simulink model "SolarTrackerHardwareModel"  (R2020a)
settings: Solver=FixedStepAuto  StartTime=0.0  StopTime=10.0  RelTol=1e-3
undefined symbols (not defined in the file): Fi, Wi
libraries: arduinowifilib x5, arduinolib x2, simulink x2
settings Model: SILPILModeSetting=veronly  ExtModeTrigDuration=2  Creator=cstap  LastModifiedBy=cstapels
settings OptimizationCC: EnhancedBackFolding=on  PassReuseOutputArgsAs=Individual arguments  ZeroExternalMemoryAtStartup=off  ZeroInternalMemoryAtStartup=off  MaxStackSize=64  OptimizeBlockOrder=speed  DifferentSizesBufferReuse=on  OptimizationCustomize=off  EfficientTunableParamExpr=on
settings DebuggingCC: ParameterTunabilityLossMsg=error
settings HardwareCC: ProdBitPerPointer=32  ProdBitPerSizeT=32  ProdBitPerPtrDiffT=32  ProdLargestAtomicInteger=Long  ProdLargestAtomicFloat=Double  ProdWordSize=32  ProdHWDeviceType=ARM Compatible->ARM Cortex
settings SFSimCC: MATLABDynamicMemAlloc=off
settings RTWCC: SystemTargetFile=ert.tlc  HardwareBoard=Arduino MKR1000  TLCOptions=-aInlineSetEventsForThisBaseRateFcn=TLC_FALSE -aSuppressMultiTaskScheduler=TLC_FALSE -aRateBasedStepFcn=1  TemplateMakefile=ert_default_tmf  Toolchain=Arduino ARM  BuildConfiguration=Faster Runs
settings CodeAppCC: ForceParamTrailComments=on  IgnoreCustomStorageClasses=off  OperatorAnnotations=on  SimulinkDataObjDesc=on  SFDataObjDesc=on  InsertBlockDesc=on
settings ERTTargetCC: SupportContinuousTime=on  SupportVariableSizeSignals=on  ExtModeStaticAllocSize=8192

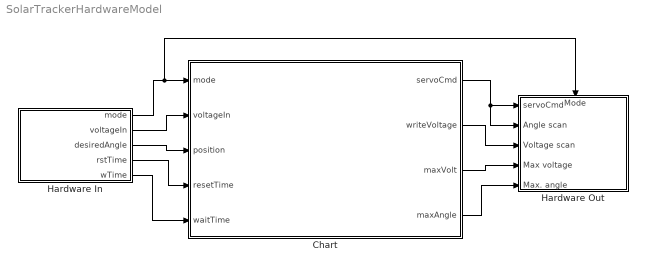
== system SolarTrackerHardwareModel ==
  Chart : Stateflow chart  TreatAsAtomicUnit=on
      settings: PortSchema="{\"entries\":[{\"content\":{\"sides\":[{\"content\":{\"connectorIds\":[\"In5\",\"In1\",\"In2\",\"In3\",\"In4\"]},\"type\":\"ConnectorPlacement.EquallySpacedRectSide\",\"uuid\":\"7460febf-f6e8-4dab-9ef6-8acf957c7b17\"},{\"content\":{\"connectorIds\":[\"Out1\",\"Out2\",\"Out3\",\"Out4\"],\"side\":\"RIGHT\"},\"type\":\"ConnectorPlacement.EquallySpacedRectSide\",\"uuid\":\"34f4fde0-3abd-4f83-b5ac-d115b7860e10\"},{\"content\":{\"connectorIds\":[],\"side\":\"TOP\"},\"type\":\"ConnectorPlacement.EquallySpacedRectSide\",\"uuid\":\"03c52414-b361-422d-a974-9760757eaedc\"}]},\"type\":\"ConnectorPlacement.EquallySpacedConnector\",\"uuid\":\"cf5b2fd0-3883-4494-a5b1-8c312db57bd7\"}],\"packageUris\":[\"http://schema.mathworks.com/mf0/Connector/19700101\"],\"version\":\"1.0\"}"
  Hardware In : Subsystem  VariantControl=simulationMode == 0
  Hardware Out : Subsystem  VariantControl=simulationMode == 0
      settings: PortSchema="{\"entries\":[{\"content\":{\"sides\":[{\"content\":{\"connectorIds\":[\"In1\",\"In2\",\"In3\",\"In4\",\"In5\"]},\"type\":\"ConnectorPlacement.EquallySpacedRectSide\",\"uuid\":\"deada059-bee1-4c5a-83e8-1a3ffab69375\"},{\"content\":{\"connectorIds\":[],\"side\":\"RIGHT\"},\"type\":\"ConnectorPlacement.EquallySpacedRectSide\",\"uuid\":\"cbd49981-471a-4624-8e3d-3b37af600932\"},{\"content\":{\"connectorIds\":[\"In6\"],\"side\":\"TOP\"},\"type\":\"ConnectorPlacement.EquallySpacedRectSide\",\"uuid\":\"9a45ed85-a60b-4cc5-836b-a1fc991137ba\"}]},\"type\":\"ConnectorPlacement.EquallySpacedConnector\",\"uuid\":\"2ce86ef1-c832-4a6c-ba54-7fb04718268c\"}],\"packageUris\":[\"http://schema.mathworks.com/mf0/Connector/19700101\"],\"version\":\"1.0\"}"
  wires:
  Hardware In/1(mode) -> Hardware Out/6(Mode), Chart/5(mode)
  Hardware In/2(voltageIn) -> Chart/1(voltageIn)
  Hardware In/3(desiredAngle) -> Chart/2(position)
  Hardware In/4(rstTime) -> Chart/3(resetTime)
  Hardware In/5(wTime) -> Chart/4(waitTime)
  Chart/1(servoCmd) -> Hardware Out/2(Angle scan), Hardware Out/1(servoCmd)
  Chart/2(writeVoltage) -> Hardware Out/3(Voltage scan)
  Chart/3(maxVolt) -> Hardware Out/4(Max voltage)
  Chart/4(maxAngle) -> Hardware Out/5(Max. angle)

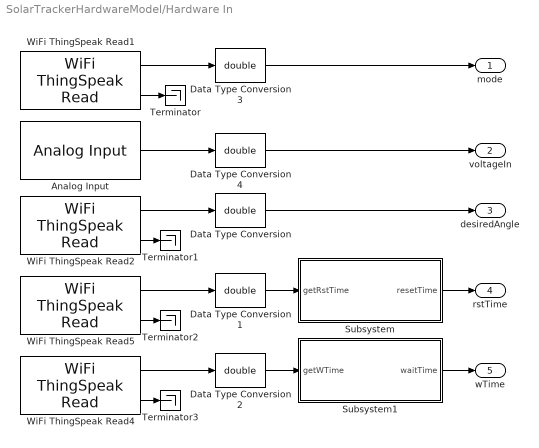
== system SolarTrackerHardwareModel/Hardware In ==
  Analog Input : arduinolib/Analog Input  pinNumber=1  ReadResultsOnly=off  ConversionTriggerSource=Software  ExternalTriggerType=uint32( 0 )  OutputDataType=uint16  EnableConversionCompleteNotify=off  EnableOuputStatus=off  SampleTime=-1  blockPlatform=arduino
  Data Type Conversion{,1..4} (5 alike) : DataTypeConversion  OutDataTypeStr=double
  Subsystem : Subsystem
  Subsystem1 : Subsystem
  Terminator{,1..3} (4 alike) : Terminator
  WiFi ThingSpeak Read1 : arduinowifilib/WiFi ThingSpeak Read  ChannelID_=1005403  ChannelAccess_=Private  ReadAPIKey_=RTAKGVYMGG3OII72  FieldNumber_=1  PrintDiagnosticMessages_=off  blockPlatform=Arduino  Interfacetype_=Wi-Fi  SampleTime_=30
      settings: SourceProductBaseCode=ARDUINO
  WiFi ThingSpeak Read2 : arduinowifilib/WiFi ThingSpeak Read  ChannelID_=1005403  ChannelAccess_=Private  ReadAPIKey_=RTAKGVYMGG3OII72  FieldNumber_=2  PrintDiagnosticMessages_=off  blockPlatform=Arduino  Interfacetype_=Wi-Fi  SampleTime_=30
      settings: SourceProductBaseCode=ARDUINO
  WiFi ThingSpeak Read4 : arduinowifilib/WiFi ThingSpeak Read  ChannelID_=1005403  ChannelAccess_=Private  ReadAPIKey_=RTAKGVYMGG3OII72  FieldNumber_=4  PrintDiagnosticMessages_=off  blockPlatform=Arduino  Interfacetype_=Wi-Fi  SampleTime_=30
      settings: SourceProductBaseCode=ARDUINO
  WiFi ThingSpeak Read5 : arduinowifilib/WiFi ThingSpeak Read  ChannelID_=1005403  ChannelAccess_=Private  ReadAPIKey_=RTAKGVYMGG3OII72  FieldNumber_=3  PrintDiagnosticMessages_=off  blockPlatform=Arduino  Interfacetype_=Wi-Fi  SampleTime_=30
      settings: SourceProductBaseCode=ARDUINO
  mode : Outport
  voltageIn : Outport  Port=2
  desiredAngle : Outport  Port=3
  rstTime : Outport  Port=4
  wTime : Outport  Port=5
  wires:
  WiFi ThingSpeak Read1/2 -> Terminator/1
  Subsystem/1(resetTime) -> rstTime/1
  Subsystem1/1(waitTime) -> wTime/1
  Analog Input/1 -> Data Type Conversion4/1
  WiFi ThingSpeak Read1/1 -> Data Type Conversion3/1
  Data Type Conversion/1 -> desiredAngle/1
  Data Type Conversion1/1 -> Subsystem/1(getRstTime)
  Data Type Conversion2/1 -> Subsystem1/1(getWTime)
  WiFi ThingSpeak Read2/1 -> Data Type Conversion/1
  WiFi ThingSpeak Read2/2 -> Terminator1/1
  WiFi ThingSpeak Read4/2 -> Terminator3/1
  WiFi ThingSpeak Read4/1 -> Data Type Conversion2/1
  WiFi ThingSpeak Read5/1 -> Data Type Conversion1/1
  WiFi ThingSpeak Read5/2 -> Terminator2/1
  Data Type Conversion3/1 -> mode/1
  Data Type Conversion4/1 -> voltageIn/1

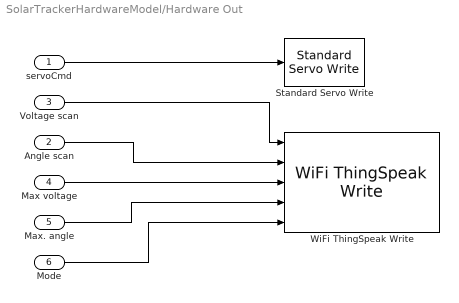
== system SolarTrackerHardwareModel/Hardware Out ==
  servoCmd : Inport
  Angle scan : Inport  Port=2
  Voltage scan : Inport  Port=3
  Max voltage : Inport  Port=4
  Max. angle : Inport  Port=5
  Mode : Inport  Port=6
  Standard Servo Write : arduinolib/Standard Servo Write  pinNumber=9  ServoIndex=0  blockPlatform=ARDUINO
  WiFi ThingSpeak Write : arduinowifilib/WiFi ThingSpeak Write  ChannelID_=1049171  WriteAPIKey_=MXTVN2YNFBXXKHG7  NumberOfFields=5  UpdateInterval_=3  PrintDiagnosticMessages_=off  LocationEnabled=off  LocationSource=Block dialog  blockPlatform=arduino  Interfacetype_=Wi-Fi  UpdateURL=0  StatusMessage=0  StatusEnabled=on  StatusSource=<empty>
      settings: SourceProductBaseCode=ARDUINO
  wires:
  Max voltage/1 -> WiFi ThingSpeak Write/3
  Max. angle/1 -> WiFi ThingSpeak Write/4
  Mode/1 -> WiFi ThingSpeak Write/5
  Angle scan/1 -> WiFi ThingSpeak Write/2
  servoCmd/1 -> Standard Servo Write/1
  Voltage scan/1 -> WiFi ThingSpeak Write/1

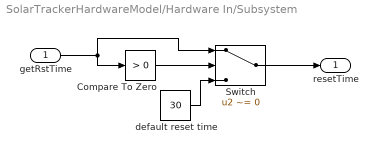
== system SolarTrackerHardwareModel/Hardware In/Subsystem ==
  getRstTime : Inport  OutDataTypeStr=double
  Compare To Zero : simulink/Logic and Bit Operations/Compare To Zero  relop=>  OutDataTypeStr=boolean
  Switch : Switch  Criteria=u2 ~= 0
  default reset time : Constant  Value=30  SampleTime=-1
  resetTime : Outport  OutDataTypeStr=double
  wires:
  Compare To Zero/1 -> Switch/2
  default reset time/1 -> Switch/3
  getRstTime/1 -> Switch/1, Compare To Zero/1
  Switch/1 -> resetTime/1

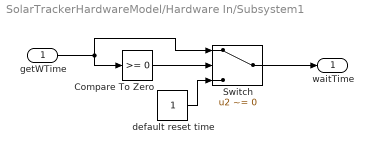
== system SolarTrackerHardwareModel/Hardware In/Subsystem1 ==
  getWTime : Inport  OutDataTypeStr=double
  Compare To Zero : simulink/Logic and Bit Operations/Compare To Zero  relop=>=  OutDataTypeStr=boolean
  Switch : Switch  Criteria=u2 ~= 0  OutDataTypeStr=double
  default reset time : Constant  SampleTime=-1
  waitTime : Outport  OutDataTypeStr=double
  wires:
  Compare To Zero/1 -> Switch/2
  default reset time/1 -> Switch/3
  getWTime/1 -> Switch/1, Compare To Zero/1
  Switch/1 -> waitTime/1

== stateflow chart SolarTrackerHardwareModel/Chart ==
  settings: updateMethod=DISCRETE  sampleTime=0.1
  state GoToPosition
    servoCmd = position;
    writeVoltage=voltageIn;
  state ScanAndGoToMaxVoltage
    state ResetPosition
      servoCmd = 0;
      voltage = zeros(1,181);
    state ScanVoltages
      servoCmd = angleRange(i);
      voltage(i) = voltageIn;
      writeVoltage = voltage(i);
    state Increment
      entry: i = i + 5;
    state GoToMaxVoltage
      [maxVolt,maxVoltAngle] = max(voltage);
      servoCmd = angleRange(maxVoltAngle);
      maxAngle = servoCmd;
      writeVoltage=voltageIn;
    (default) -> ResetPosition : {angleRange = 0 :180;}
    GoToMaxVoltage -> ResetPosition : after(resetTime,sec)
    ResetPosition -> ScanVoltages : {i = 1;}
    ScanVoltages -> Increment [order 1] : [i < 181]
    Increment -> ScanVoltages : after(waitTime,msec)
    ScanVoltages -> GoToMaxVoltage [order 2] : [i==181]
  (default) -> GoToPosition
  GoToPosition -> ScanAndGoToMaxVoltage : [mode==1]
  ScanAndGoToMaxVoltage -> GoToPosition : [mode==0]
  data: voltageIn input; position input; servoCmd output; writeVoltage output; maxVolt output; maxAngle output; voltage local; i local; maxVoltAngle local; resetTime input; waitTime input; mode input; angleRange local
